simulink model "testARINC"  (R2021b)
settings: Solver=FixedStepDiscrete  StartTime=0.0  StopTime=10.0  FixedStep=1e-3  RelTol=1e-3
undefined symbols (not defined in the file): IO682
libraries: speedgoatlib_IO682 x5
settings Model: Creator=ACH  LastModifiedBy=ACH

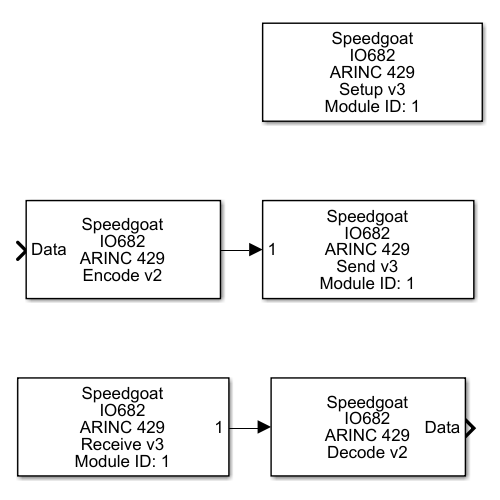
[thumbnail: Simulink's stored preview of the top-level diagram]
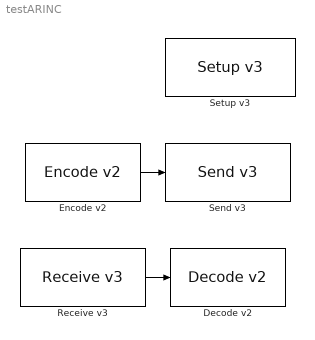
== system testARINC ==
  "Decode v2 " : speedgoatlib_IO682/Decode v2   parMode=Standard  parLabel=[002]  parDataType=[1]  parResolution=[1]  parSyncMask=hex2dec('0x0')  parSyncValue=hex2dec('0x0')  parCustomDataType=Raw  parDataLSB=9  parDataMSB=31  parBitPosition=[9, 31]  parScaleBNR=1  parExponent=8  parMantissa=14  parTimeTags=off  parHoldLastVal=on  parStatus=off
      settings: SourceProductName=Simulink Real-Time: Speedgoat I/O Blockset
  "Encode v2 " : speedgoatlib_IO682/Encode v2   parMode=Standard  parLabel=[002]  parDataType=[1]  parResolution=[1]  parBits=[19]  parSdi=[0]  parSsm=[-1]  parCustomDataType=Raw  parDataLSB=9  parDataMSB=31  parBitPosition=[9, 31]  parScaleBNR=1  parExponent=8  parMantissa=14  parEnSSM=off
      settings: SourceProductName=Simulink Real-Time: Speedgoat I/O Blockset
  "Receive v3 " : speedgoatlib_IO682/Receive v3   parModuleId=1  parChannel=1  parMaxWords=50  parMinWords=1  parSampleTime=-1
      settings: SourceProductName=Simulink Real-Time: Speedgoat I/O Blockset
  "Send v3 " : speedgoatlib_IO682/Send v3   parModuleId=1  parChannel=1  parSampleTime=-1
      settings: SourceProductName=Simulink Real-Time: Speedgoat I/O Blockset
  "Setup v3 " : speedgoatlib_IO682/Setup v3   parModuleId=1  parBoardVariant=IO682-2-2  parPciSlot=-1  parTimerCount=4000  parChannelMode=Manual  parInBitRate1=100000  parInBufferMode1=Individual  parInEnable1=on  parInParity1=on  parInInternalWrap1=off  parInBitRate2=100000  parInBufferMode2=Individual  parInEnable2=on  parInParity2=on  parInInternalWrap2=off  parInBitRate3=100000  parInBufferMode3=Individual  parInEnable3=on  parInParity3=on  parInInternalWrap3=off  parInBitRate4=100000  parInBufferMode4=Individual  parInEnable4=on  parInParity4=on  parInInternalWrap4=off  parInBitRate5=100000  parInBufferMode5=Individual  parInEnable5=on  parInParity5=on  parInInternalWrap5=off  parInBitRate6=100000  parInBufferMode6=Individual  parInEnable6=on  parInParity6=on  parInInternalWrap6=off  parInBitRate7=100000  parInBufferMode7=Individual  parInEnable7=on  parInParity7=on  parInInternalWrap7=off  parInBitRate8=100000  parInBufferMode8=Individual  parInEnable8=on  parInParity8=on  parInInternalWrap8=off  parInBitRate9=100000  parInBufferMode9=Individual  parInEnable9=on  parInParity9=on  parInInternalWrap9=off  parInBitRate10=100000  parInBufferMode10=Individual  parInEnable10=on  parInParity10=on  parInInternalWrap10=off  parInBitRate11=100000  parInBufferMode11=Individual  parInEnable11=on  parInParity11=on  parInInternalWrap11=off  parInBitRate12=100000  parInBufferMode12=Individual  parInEnable12=on  parInParity12=on  parInInternalWrap12=off  parInBitRate13=100000  parInBufferMode13=Individual  parInEnable13=on  parInParity13=on  parInInternalWrap13=off  parInBitRate14=100000  parInBufferMode14=Individual  parInEnable14=on  parInParity14=on  parInInternalWrap14=off  parInBitRate15=100000  parInBufferMode15=Individual  parInEnable15=on  parInParity15=on  parInInternalWrap15=off  parInBitRate16=100000  parInBufferMode16=Individual  parInEnable16=on  parInParity16=on  parInInternalWrap16=off  parOutBitRate1=100000  parOutParity1=Odd  parOutProtocolError1=None  parOutEnable1=on  parOutBitRate2=100000  parOutParity2=Odd  parOutProtocolError2=None  parOutEnable2=on  parOutBitRate3=100000  parOutParity3=Odd  parOutProtocolError3=None  parOutEnable3=on  parOutBitRate4=100000  parOutParity4=Odd  parOutProtocolError4=None  parOutEnable4=on  parOutBitRate5=100000  parOutParity5=Odd  parOutProtocolError5=None  parOutEnable5=on  parOutBitRate6=100000  parOutParity6=Odd  parOutProtocolError6=None  parOutEnable6=on  parOutBitRate7=100000  parOutParity7=Odd  parOutProtocolError7=None  parOutEnable7=on  parOutBitRate8=100000  parOutParity8=Odd  parOutProtocolError8=None  parOutEnable8=on  parOutBitRate9=100000  parOutParity9=Odd  parOutProtocolError9=None  parOutEnable9=on  parOutBitRate10=100000  parOutParity10=Odd  parOutProtocolError10=None  parOutEnable10=on  parOutBitRate11=100000  parOutParity11=Odd  parOutProtocolError11=None  parOutEnable11=on  parOutBitRate12=100000  parOutParity12=Odd  parOutProtocolError12=None  parOutEnable12=on  parOutBitRate13=100000  parOutParity13=Odd  parOutProtocolError13=None  parOutEnable13=on  parOutBitRate14=100000  parOutParity14=Odd  parOutProtocolError14=None  parOutEnable14=on  parOutBitRate15=100000  parOutParity15=Odd  parOutProtocolError15=None  parOutEnable15=on  parOutBitRate16=100000  parOutParity16=Odd  parOutProtocolError16=None  parOutEnable16=on  parChConfigFile=''  parScheduleMode=Manual  parScheduledMsgConfigFile=''  parHwDeviceId=hex2dec('0830')  parTimeSource=Internal timer  parChInConfig=[158 8 7 7 1;158 8 7 7 1]  parChOutConfig=[158 0 4 7;158 0 4 7]  parScheduledMessages=0
      settings: SourceProductName=Simulink Real-Time: Speedgoat I/O Blockset
  wires:
  "Encode v2 "/1 -> "Send v3 "/1
  "Receive v3 "/1 -> "Decode v2 "/1
